simulink model "Trial2"  (R2020b)
settings: Solver=VariableStepAuto  StartTime=0.0  StopTime=100  RelTol=1e-3
values from neighbouring files (symbols this model uses):
  A_AD = horzcat(A_i, A_ii)    [six.m]
  A_kal = [0 0 0 1 0 0 ... (first row only)    [six.m]
  B_AD = horzcat(B_i, B_ii)    [six.m]
  B_kal = [0 0 0 0 0 0 ... (first row only)    [six.m]
  C_AD = eye(6)    [six.m]
  C_D = 0.2    [Point_Mass.m]    (also in Point_mass_fancy_results.m = 0.6; point_mass_MAIN.m = 0.02; point_mass_unit_test_func.m = C_D; point_mass_verification.m)
  C_kal = eye(6)    [six.m]
  D_AD = zeros(6)    [six.m]
  D_kal = zeros(6)    [six.m]
  g = theta_dd_0*theta_d_0*cos(theta_0)*I_xy - phi_d_0*(theta_d_0)^2*sin(theta_0)*I_xy - phi_dd_0*theta_d_0*sin(theta_0)*I_xz - theta_d_0^2 * cos(theta_0)*I_xz + phi_d_0 * I_zx * theta_d_0 * cos(theta_0) + I_zy*phi_d_0^2*theta_d_0*sin(2*theta_0) + I_zz*phi_d_0 * theta_d_0 * cos(2*theta_0) + phi_d_0 * theta_d_0 * I_yx * sin(theta_0) - phi_d_0^2 * I_yy * theta_d_0 * cos(2*theta_0) + phi_d_0^2 * theta_d_0  ...(+23 chars)    [Gyro.m]    (also in Point_Mass.m = 9.81; Point_mass_fancy_results.m = 9.81; Tdt.m = cos(phi)*sin(theta)*cos(psi) + sin(phi)*sin(psi); angular_tune.m = (I_yx*I_zy - I_yy*I_zx)*(I_zx*wy_0 - I_yx*wz_0) + (I_xy*I_zx)
  m = theta_d_0*cos(theta_0)*I_yy - theta_d_0*sin(theta_0)*I_yz + I_xx*cos(theta_0)*theta_d_0 + 2*phi_d_0*I_xy*cos(theta_0)*sin(theta_0) + 2*phi_d_0*I_xz*(cos(theta_0))^2 - theta_d_0 * I_zy * sin(theta_0) - theta_d_0*cos(theta_0)*I_zz    [Gyro.m]    (also in Point_Mass.m = 100; Point_mass_fancy_results.m = 600; point_mass_MAIN.m = 640; point_mass_unit_test_func.m = mass)
  rho = 0.991    [Point_Mass.m]    (also in Point_mass_fancy_results.m = 1.225; point_mass_MAIN.m = 1.225; point_mass_unit_test_func.m = density; point_mass_verification.m = 1.225)
  S = 4.5    [Point_Mass.m]    (also in Point_mass_fancy_results.m = 1.8; point_mass_MAIN.m = 2; point_mass_unit_test_func.m = S; point_mass_verification.m = 2)
  T = 10.5    [Point_mass_fancy_results.m]    (also in point_mass_MAIN.m; point_mass_unit_test_func.m = T; point_mass_verification.m = 1.5; six.m)
  time_delay = 0.3    [Point_mass_fancy_results.m]    (also in point_mass_MAIN.m = 3e-05; point_mass_unit_test_func.m = time_delay; point_mass_verification.m = 0.1; six.m = 0.1)
  w_0 = [0;0;0]    [Propellers_tilt.m]    (also in six.m; tilt_verification.m)
undefined symbols (not defined in the file or in its folder): A_2, B_2, C_2, Continuous, D_2, Fb1_l, Fb1_u, Fb2_l, Fb2_u, Fb3_l, Fb3_u, Fb4_l, Fb4_u, Fc1_l, Fc1_u, Fc2_l, Fc2_u, Fc3_l, Fc3_u, Ft1_l, Ft1_u, Ft2_l, Ft2_u, Ft3_l, Ft3_u, Ft4_l, Ft4_u, r_0, Time, v_0, ZI_Cx, ZI_Cy, ZI_Cz, ZI_p, ZI_q, ZI_r
libraries: pid_lib x3, dspsigops x3, fuzblock x3, dspindex x3, ctrlSharedLib x2, simulink x1, mpclib x1, dspmathops x1, cstblocks x1
(part 2 of 2)

== matlab function Trial2/Transformation Subsystem/MATLAB Function2 ==
  data: theta_x input; Transformation_Mat output; theta_y input; theta_z input
function Transformation_Mat  = Euler(theta_x, theta_y, theta_z)

a = cos(theta_x)*cos(theta_z);
b = cos(theta_x)*sin(theta_z);
c = - sin(theta_x);
d = sin(theta_y)*sin(theta_x)*cos(theta_z) - cos(theta_y)*sin(theta_z);
e = sin(theta_y)*sin(theta_x)*sin(theta_z) + cos(theta_y)*cos(theta_z);
f = sin(theta_y)*cos(theta_x);
g = cos(theta_y)*sin(theta_x)*cos(theta_z) + sin(theta_y)*sin(theta_z);
h = cos(theta_y)*sin(theta_x)*sin(theta_z) - sin(theta_y)*cos(theta_z);
i = cos(theta_y)*cos(theta_x);

Transformation_Mat = [a b c;
    d e f;
    g h i];


end

== matlab function Trial2/GPS model/GPS Model ==
  settings: updateMethod=DISCRETE
  data: position input; newposition output
function newposition  = gps(position)

    % Input: position
    % Output: position with gps accuracies inclduded
    mu = 0; 
    sigma = 0.015;

    r1 = normrnd(mu, sigma);
    r2 = normrnd(mu, sigma);
    r3 = normrnd(mu, sigma);

    newposition = [0,0,0];

    newposition(1) = position(1) + r1;
    newposition(2) = position(2) + r2;
    newposition(3) = position(3) + r3;

end

== matlab function Trial2/Transformation Subsystem/MATLAB Function1 ==
  data: theta_x input; Transformation_Mat output; theta_y input; theta_z input
function Transformation_Mat  = Euler(theta_x, theta_y, theta_z)

a = cos(theta_x)*cos(theta_z);
b = cos(theta_x)*sin(theta_z);
c = - sin(theta_x);
d = sin(theta_y)*sin(theta_x)*cos(theta_z) - cos(theta_y)*sin(theta_z);
e = sin(theta_y)*sin(theta_x)*sin(theta_z) + cos(theta_y)*cos(theta_z);
f = sin(theta_y)*cos(theta_x);
g = cos(theta_y)*sin(theta_x)*cos(theta_z) + sin(theta_y)*sin(theta_z);
h = cos(theta_y)*sin(theta_x)*sin(theta_z) - sin(theta_y)*cos(theta_z);
i = cos(theta_y)*cos(theta_x);

Transformation_Mat = [a b c;
    d e f;
    g h i];


end

== matlab function Trial2/Propulsion commands module/Propeller firing function/MATLAB Function ==
  data: F_wanted input; F_c output; M_wanted input; F_t output; F_b output
function [F_c, F_t, F_b] = propeller_required_forces_control(F_wanted, M_wanted)

%% Load propeller arms data
xc_1 = 0.1;
yc_1 = 0;
zc_1 = 0.3;
xc_2 = 0.1;
yc_2 = 0;
zc_2 = 0.32;
xc_3 = 0.11;
yc_3 = 0;
zc_3 = 0.31;

xt_1 = 0.2;
yt_1 = 0.2;
zt_1 = 1;
xt_2 = 0.2;
yt_2 = 0.2;
zt_2 = 1;
xt_3 = 0.2;
yt_3 = 0.2;
zt_3 = 1;
xt_4 = 0.2;
yt_4 = 0.2;
zt_4 = 1;

xb_1 = 0.4;
yb_1 = 0.3;
zb_1 = 1.2;
xb_2 = 0.4;
yb_2 = 0.3;
zb_2 = 1.2;
xb_3 = 0.4;
yb_3 = 0.3;
zb_3 = 1.2;
xb_4 = 0.4;
yb_4 = 0.3;
zb_4 = 1.2;

%% Decompose force and moment input

F_x = F_wanted(1);
F_y = F_wanted(2);
F_z = F_wanted(3);

M_x = M_wanted(1);
M_y = M_wanted(2);
M_z = M_wanted(3);

%% Find control forces
A_control = [1 1 1;
    zc_1 -zc_2 -zc_3;
    -xc_1 -xc_2 xc_3];
A_cinv = inv(A_control);
force_control = [F_y; M_x; M_z];
controlvec = A_cinv*force_control;
F_c1 = controlvec(1);
F_c2 = controlvec(2);
F_c3 = controlvec(3);

%% Find top and bottom forces
A_tb = [-1 -1;
    2*(xt_1 + xb_1) -2*(xt_3 + xb_3)];
A_tbinv = inv(A_tb);
force_tb = [F_z; M_y];
tbvec = A_tbinv * force_tb;
f_front = tbvec(1);
F_t1 = f_front/4;
F_t2 = f_front/4;
F_b1 = f_front/4;
F_b2 = f_front/4;
f_back = tbvec(2);
F_t3 = f_back/4;
F_t4 = f_back/4;
F_b3 = f_back/4;
F_b4 = f_back/4;



%% Make matrix
F_c = [F_c1; F_c2; F_c3];
F_t = [F_t1; F_t2; F_t3; F_t4];
F_b = [F_b1; F_b2; F_b3; F_b4];
end

== matlab function Trial2/Subsystem2/MATLAB Function ==
  settings: updateMethod=DISCRETE
  data: angvel input; accelData output; acc input
function accelData = accelerometer(angvel, acc)

    %
    % Create gyroscope sensor object
    params = accelparams;
    
    % Parameters for simulated signal
    N = 1;       % Number of samples
    Fs = 100000;       % Sampling rate
    %Fc = 0.25;      % Sinusoidal frequency
    
    
    % Create arrays
    t = (0:(1/Fs):((N-1)/Fs)).';
    acc = acc;          %Input accelerations
    orient = quaternion.ones(N, 1);
    angvel = angvel;
    
    % Generate acceleration data
    imu = imuSensor('SampleRate', Fs, 'Accelerometer', params);
    imu.Accelerometer.MeasurementRange = 1000;   % Maximum acceleration accelerometer can measure
    imu.Accelerometer.Resolution = 1/Fs;           % Step size of digital measurements
    
    % Biases
    imu.Accelerometer.BiasInstability = 0.000000000001; 7.5 / 1000 * 9.81;
    imu.Accelerometer.NoiseDensity = 0.000000000001;%150 / 1000 / 1000 * 9.81 /10; 
    imu.Accelerometer.TemperatureBias = 50 / 1000 / 1000 * 9.81;
    
  
    
    accelData = imu(acc, angvel, orient);
    
    accelData(:,3) = accelData(:,3) - 9.81;

    accelData(:,1) = accelData(:,1) * -1;
    accelData(:,2) = accelData(:,2) * -1;
    accelData(:,3) = accelData(:,3) * -1;

end

== matlab function Trial2/Gyroscope Model/MATLAB Function ==
  settings: updateMethod=DISCRETE
  data: xvel input; yvel input; zvel input; gyroData output; acc input
function gyroData  = fungyroscope(xvel, yvel, zvel, acc)
   
    % Create gyroscope sensor object
    params = gyroparams;         
    
    % Parameters for simulated signal
    N = 1;       % Number of samples
    Fs = 100;       % Sampling rate
    Fc = 0.25;      % Sinusoidal frequency
    
    % Create arrays
    t = (0:(1/Fs):((N-1)/Fs)).';
    acc = acc;          % Input accelerations
    angvel = [xvel,yvel,zvel];
    %angvel(:,1) = 8*sin(2*pi*Fc*t);
    
    % Generate gyroscopic data
    imu = imuSensor('SampleRate', Fs, 'Gyroscope', params);
    imu.Gyroscope.MeasurementRange = 6.5;   % Maximum angular velocity gyroscope can measure
    imu.Gyroscope.Resolution = 1/Fs;           % Step size of digital measurements
    
    % Biases
    
    imu.Gyroscope.BiasInstability = 0.12 * 3.14159 / 180;       % rad/hr
    imu.Gyroscope.NoiseDensity = 0.15 * 3.14159 / 180;          % rad/s
    imu.Gyroscope.RandomWalk = 0.017 * 3.14159 / 180;           % rad/sqrt(hr)
    imu.Gyroscope.TemperatureBias = 0.25 * 3.14159 / 180;       % rad/s
    %imu.Gyroscope.AccelerationBias = 0.3;
    
    % Define real accelerations
    %acc(:,1) = 1;
    [~, gyroData] = imu(acc, angvel, eye(3));
    

end

== matlab function Trial2/Propulsion commands module/Subsystem3/MATLAB Function ==
  data: Fc input; Fx_acc output; Ft input; Fb input; Fy_acc output; Fz_acc output; Mx_acc output; My_acc output; Mz_acc output
function [Fx_acc,Fy_acc, Fz_acc, Mx_acc, My_acc, Mz_acc] = fcn(Fc, Ft, Fb)

%% Load propeller arms data
xc_1 = 0.1;
yc_1 = 0;
zc_1 = 0.3;
xc_2 = 0.1;
yc_2 = 0;
zc_2 = 0.32;
xc_3 = 0.11;
yc_3 = 0;
zc_3 = 0.31;

xt_1 = 0.2;
yt_1 = 0.2;
zt_1 = 1;
xt_2 = 0.2;
yt_2 = 0.2;
zt_2 = 1;
xt_3 = 0.2;
yt_3 = 0.2;
zt_3 = 1;
xt_4 = 0.2;
yt_4 = 0.2;
zt_4 = 1;

xb_1 = 0.4;
yb_1 = 0.3;
zb_1 = 1.2;
xb_2 = 0.4;
yb_2 = 0.3;
zb_2 = 1.2;
xb_3 = 0.4;
yb_3 = 0.3;
zb_3 = 1.2;
xb_4 = 0.4;
yb_4 = 0.3;
zb_4 = 1.2;


%% Split vectors
Fx_acc = 0;

A_control = [1 1 1;
    zc_1 -zc_2 -zc_3;
    -xc_1 -xc_2 xc_3];
ab_control = A_control*Fc;
Fy_acc = ab_control(1);
Mx_acc = ab_control(2);
Mz_acc = ab_control(3);

A_tb = [-1 -1;
    2*(xt_1 + xb_1) -2*(xt_3 + xb_3)];
F_front = Ft(1) + Ft(2) + Fb(1) + Fb(2);
F_back = Ft(3) + Ft(4) + Fb(3) + Fb(4);
Ftb_vec = [F_front; F_back];
Ab_tb = A_tb*Ftb_vec;

Fz_acc = Ab_tb(1);
My_acc = Ab_tb(2);

end
